simulink model "BackStepping"  (R2018b)
settings: Solver=VariableStepAuto  StartTime=0.0  StopTime=1  FixedStep=1  RelTol=0.1
values from neighbouring files (symbols this model uses):
  jointAngle = inverseKinematic.ComputeInverseKinematic(jointAngle, endPose)    [CartesianTrajectoryGeneration.m]
  jointAngleStart = [175.0; 145.0; 178.0; 90.0; 180.0; 215.0; 260.0]    [CartesianTrajectoryGeneration.m]
  K = [[100 0 0 0 0 0 0] ... (first row only)    [BackSteppingParam.m]
  Lamda = [[1 0 0 0 0 0 0] ... (first row only)    [BackSteppingParam.m]
settings Model: Creator=olavoie  LastModifiedBy=olavoie

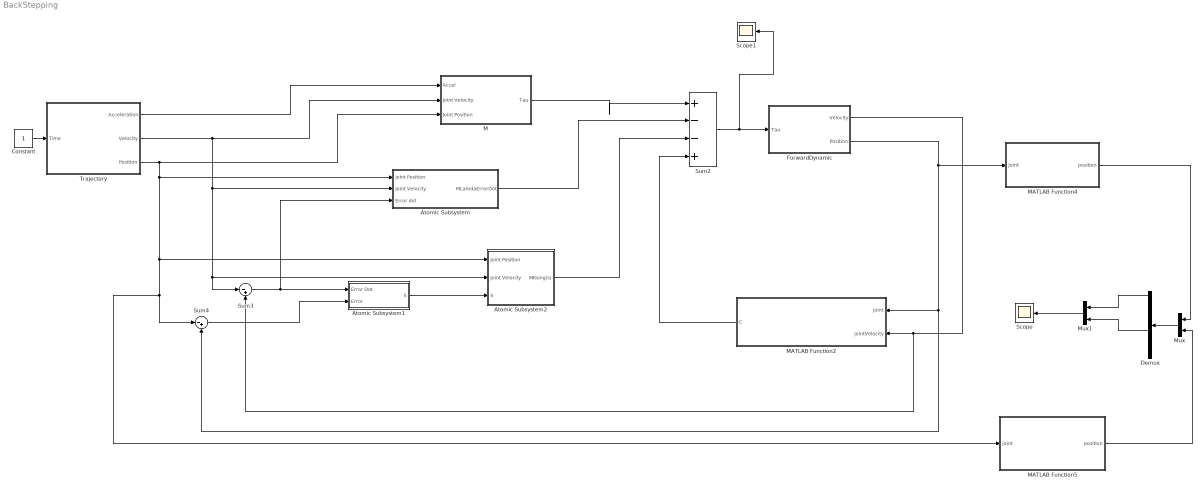
== system BackStepping ==
  Atomic Subsystem : Subsystem  TreatAsAtomicUnit=on
  Atomic Subsystem1 : Subsystem  TreatAsAtomicUnit=on
  Atomic Subsystem2 : Subsystem  TreatAsAtomicUnit=on
  Constant : Constant
  Demux : Demux  Outputs=6
  ForwardDynamic : Subsystem  TreatAsAtomicUnit=on
  M : Subsystem  TreatAsAtomicUnit=on
  MATLAB Function2 : MATLAB Function  TreatAsAtomicUnit=on
  MATLAB Function4 : MATLAB Function  TreatAsAtomicUnit=on
  MATLAB Function5 : MATLAB Function  TreatAsAtomicUnit=on
  Mux : Mux  Inputs=2
  Mux1 : Mux  Inputs=2
  Scope : Scope
  Scope1 : Scope
  Sum2 : Sum  Inputs=|+--+
  Sum3 : Sum  Inputs=|-+
  Sum4 : Sum  Inputs=|-+
  Trajectory : Subsystem  TreatAsAtomicUnit=on
  wires:
  Constant/1 -> Trajectory/1(Time)
  ForwardDynamic/1(Velocity) -> Sum3/2, MATLAB Function2/2(jointVelocity)
  Trajectory/1(Acceleration) -> M/1("Accel ")
  Trajectory/2(Velocity) -> Sum3/1, Atomic Subsystem2/2(Joint Velocity), Atomic Subsystem/2(Joint Velocity), M/2(Joint Velocity)
  Sum3/1 -> Atomic Subsystem/3(Error dot), Atomic Subsystem1/1(Error Dot)
  Sum4/1 -> Atomic Subsystem1/2(Error)
  Atomic Subsystem1/1(S) -> Atomic Subsystem2/3(S)
  Sum2/1 -> Scope1/1, ForwardDynamic/1(Tau)
  MATLAB Function2/1(C) -> Sum2/4
  M/1(Tau) -> Sum2/1
  MATLAB Function5/1(position) -> Mux/2
  MATLAB Function4/1(position) -> Mux/1
  ForwardDynamic/2(Position) -> Sum4/2, MATLAB Function2/1(joint), MATLAB Function4/1(joint)
  Trajectory/3(Position) -> Sum4/1, MATLAB Function5/1(joint), Atomic Subsystem2/1(Joint Position), Atomic Subsystem/1(Joint Position), M/3(Joint Position)
  Atomic Subsystem/1(MLamdaErrorDot) -> Sum2/2
  Atomic Subsystem2/1(MKsing(s)) -> Sum2/3
  Mux/1 -> Demux/1
  Demux/1 -> Mux1/1
  Demux/4 -> Mux1/2
  Mux1/1 -> Scope/1

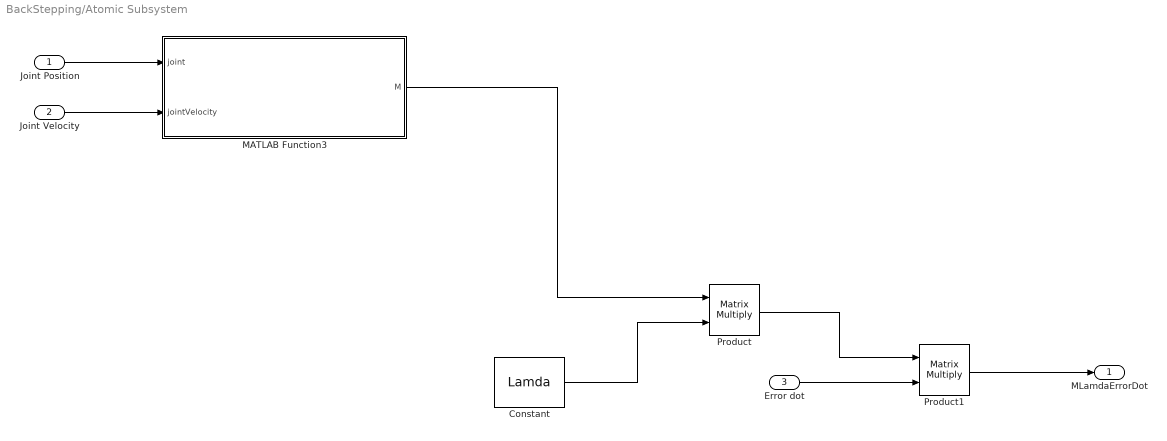
== system BackStepping/Atomic Subsystem ==
  Joint Position : Inport
  Joint Velocity : Inport  Port=2
  Error dot : Inport  Port=3
  Constant : Constant  Value=Lamda
  MATLAB Function3 : MATLAB Function  TreatAsAtomicUnit=on
  Product : Product  Multiplication=Matrix(*)
  Product1 : Product  Multiplication=Matrix(*)
  MLamdaErrorDot : Outport
  wires:
  Joint Position/1 -> MATLAB Function3/1(joint)
  Joint Velocity/1 -> MATLAB Function3/2(jointVelocity)
  Product1/1 -> MLamdaErrorDot/1
  Error dot/1 -> Product1/2
  Product/1 -> Product1/1
  Constant/1 -> Product/2
  MATLAB Function3/1(M) -> Product/1

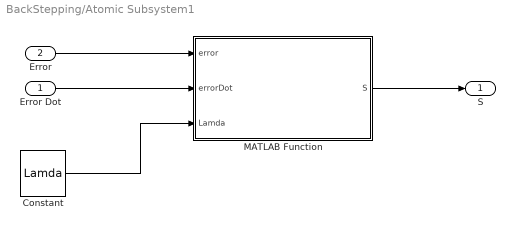
== system BackStepping/Atomic Subsystem1 ==
  Error Dot : Inport
  Error : Inport  Port=2
  Constant : Constant  Value=Lamda
  MATLAB Function : MATLAB Function  TreatAsAtomicUnit=on
  S : Outport
  wires:
  Error/1 -> MATLAB Function/1(error)
  Error Dot/1 -> MATLAB Function/2(errorDot)
  Constant/1 -> MATLAB Function/3(Lamda)
  MATLAB Function/1(S) -> S/1

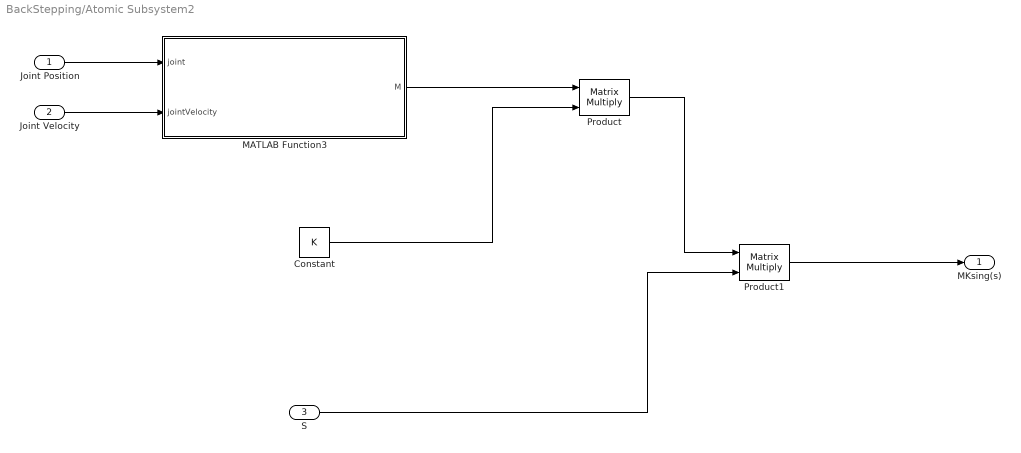
== system BackStepping/Atomic Subsystem2 ==
  Joint Position : Inport
  Joint Velocity : Inport  Port=2
  S : Inport  Port=3
  Constant : Constant  Value=K
  MATLAB Function3 : MATLAB Function  TreatAsAtomicUnit=on
  Product : Product  Multiplication=Matrix(*)
  Product1 : Product  Multiplication=Matrix(*)
  MKsing(s) : Outport
  wires:
  Joint Velocity/1 -> MATLAB Function3/2(jointVelocity)
  Joint Position/1 -> MATLAB Function3/1(joint)
  MATLAB Function3/1(M) -> Product/1
  Constant/1 -> Product/2
  Product/1 -> Product1/1
  Product1/1 -> MKsing(s)/1
  S/1 -> Product1/2

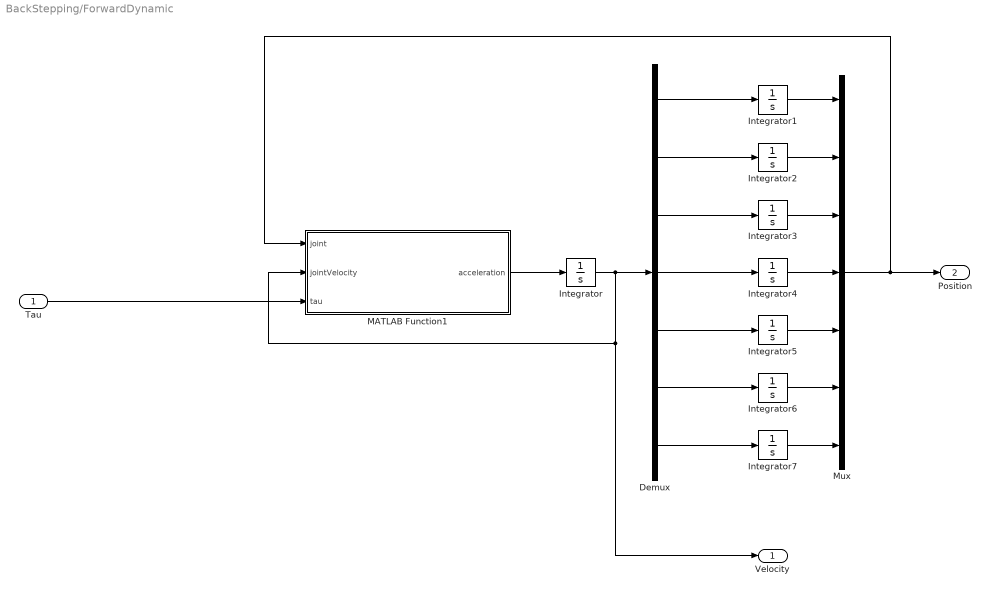
== system BackStepping/ForwardDynamic ==
  Tau : Inport
  Demux : Demux  Outputs=7
  Integrator : Integrator
  Integrator1 : Integrator  InitialCondition=jointAngleStart(1)
  Integrator2 : Integrator  InitialCondition=jointAngleStart(2)
  Integrator3 : Integrator  InitialCondition=jointAngleStart(3)
  Integrator4 : Integrator  InitialCondition=jointAngleStart(4)
  Integrator5 : Integrator  InitialCondition=jointAngleStart(5)
  Integrator6 : Integrator  InitialCondition=jointAngleStart(6)
  Integrator7 : Integrator  InitialCondition=jointAngleStart(7)
  MATLAB Function1 : MATLAB Function  TreatAsAtomicUnit=on
  Mux : Mux  Inputs=7
  Velocity : Outport
  Position : Outport  Port=2
  wires:
  Tau/1 -> MATLAB Function1/3(tau)
  MATLAB Function1/1(acceleration) -> Integrator/1
  Integrator/1 -> Velocity/1, MATLAB Function1/2(jointVelocity), Demux/1
  Demux/7 -> Integrator7/1
  Demux/6 -> Integrator6/1
  Demux/5 -> Integrator5/1
  Demux/4 -> Integrator4/1
  Demux/3 -> Integrator3/1
  Demux/1 -> Integrator1/1
  Demux/2 -> Integrator2/1
  Integrator1/1 -> Mux/1
  Integrator2/1 -> Mux/2
  Integrator3/1 -> Mux/3
  Integrator4/1 -> Mux/4
  Integrator5/1 -> Mux/5
  Integrator6/1 -> Mux/6
  Integrator7/1 -> Mux/7
  Mux/1 -> MATLAB Function1/1(joint), Position/1

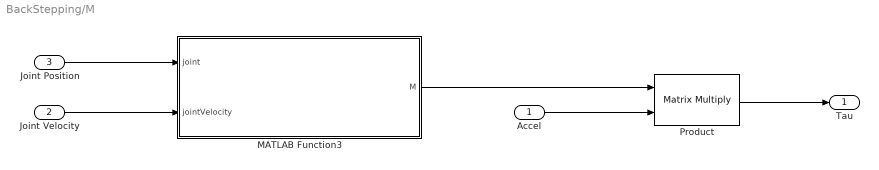
== system BackStepping/M ==
  "Accel " : Inport
  Joint Velocity : Inport  Port=2
  Joint Position : Inport  Port=3
  MATLAB Function3 : MATLAB Function  TreatAsAtomicUnit=on
  Product : Product  Multiplication=Matrix(*)
  Tau : Outport
  wires:
  MATLAB Function3/1(M) -> Product/1
  Product/1 -> Tau/1
  Joint Position/1 -> MATLAB Function3/1(joint)
  Joint Velocity/1 -> MATLAB Function3/2(jointVelocity)
  "Accel "/1 -> Product/2

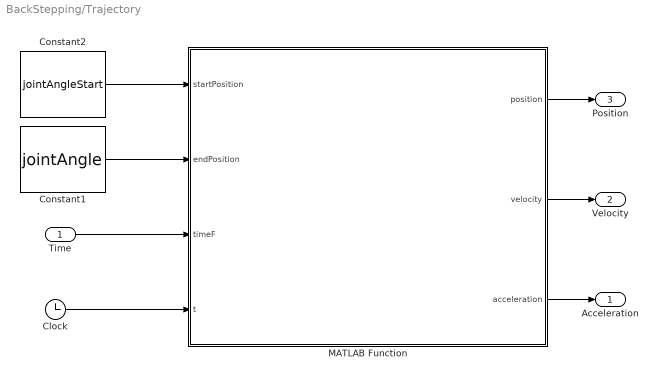
== system BackStepping/Trajectory ==
  Time : Inport
  Clock : Clock
  Constant1 : Constant  Value=jointAngle
  Constant2 : Constant  Value=jointAngleStart
  MATLAB Function : MATLAB Function  TreatAsAtomicUnit=on
  Acceleration : Outport
  Velocity : Outport  Port=2
  Position : Outport  Port=3
  wires:
  Constant1/1 -> MATLAB Function/2(endPosition)
  Time/1 -> MATLAB Function/3(timeF)
  Clock/1 -> MATLAB Function/4(t)
  Constant2/1 -> MATLAB Function/1(startPosition)
  MATLAB Function/1(position) -> Position/1
  MATLAB Function/2(velocity) -> Velocity/1
  MATLAB Function/3(acceleration) -> Acceleration/1

== matlab function BackStepping/M/MATLAB Function3 ==
  data: joint input; M output; jointVelocity input
function M = MassMatrix(joint, jointVelocity)
    % Robot Frame    
    robotData = RobotParam;
    
    % Mass Center
    Pc = zeros(3,7);
    Pc(:, 1) = [ -3.94e-06;  0.001804699;  -0.0748562];
    Pc(:, 2) = [2.2339e-05;   0.07515658;  -0.0301928];
    Pc(:, 3) = [-2.234e-05;  0.009582299;  -0.0966774];
    Pc(:, 4) = [-3.269e-05;   0.09546485;  -0.0287837];
    Pc(:, 5) = [6.4423e-05;  -0.00987523;  -0.0607337];
    Pc(:, 6) = [5.6819e-05;   0.04279498; -0.00982194];
    Pc(:, 7) = [         0;       -2e-05;    -0.01702];

    % Mass
    m = [1.290800 1.344200 1.344200 1.094520 0.590200 0.590200 0.239480];

    % Inertia
    I = zeros(3, 3,7);
    I(:, :, 1) = [101, 0, 0; 0, 101, 0; 0, 0, 101];
    I(:, :, 2) = [102, 0, 0; 0, 102, 0; 0, 0, 102];
    I(:, :, 3) = [103, 0, 0; 0, 103, 0; 0, 0, 103];
    I(:, :, 4) = [104, 0, 0; 0, 104, 0; 0, 0, 104];
    I(:, :, 5) = [105, 0, 0; 0, 105, 0; 0, 0, 105];
    I(:, :, 6) = [106, 0, 0; 0, 106, 0; 0, 0, 106];
    I(:, :, 7) = [107, 0, 0; 0, 107, 0; 0, 0, 107];

    R = zeros(3, 3, robotData.mActuatorCount + 1);
    P = zeros(3, robotData.mActuatorCount + 1);

    % Robot referential
    for n = 1:robotData.mActuatorCount
        T = robotData.mJointReferentiel(:, :, n) * rotm2tform(rotz(joint(n) + robotData.mJointOffset(n)));
        R(:, :, n) = tform2rotm(T);
        P(:, n)    = tform2trvec(T);
    end
    
    R(:, :, robotData.mActuatorCount + 1) = [1, 0, 0; 0, 1, 0; 0, 1, 0];
    P(:, robotData.mActuatorCount + 1)    = [0; 0; 0];

    C = InverseDynamicSolver(R, P, Pc, I, m, jointVelocity, [0; 0; 0; 0; 0; 0; 0; 0], robotData.mActuatorCount)';

    M = zeros(7,7);
    for n = 1:robotData.mActuatorCount
        a = [0; 0; 0; 0; 0; 0; 0];
        a(n) = 1;
        M(:, n) = InverseDynamicSolver(R, P, Pc, I, m, jointVelocity, a, robotData.mActuatorCount)' - C;
    end 
end

== matlab function BackStepping/Atomic Subsystem/MATLAB Function3 ==
  data: joint input; M output; jointVelocity input
function M = MassMatrix(joint, jointVelocity)
    % Robot Frame    
    robotData = RobotParam;
    
    % Mass Center
    Pc = zeros(3,7);
    Pc(:, 1) = [ -3.94e-06;  0.001804699;  -0.0748562];
    Pc(:, 2) = [2.2339e-05;   0.07515658;  -0.0301928];
    Pc(:, 3) = [-2.234e-05;  0.009582299;  -0.0966774];
    Pc(:, 4) = [-3.269e-05;   0.09546485;  -0.0287837];
    Pc(:, 5) = [6.4423e-05;  -0.00987523;  -0.0607337];
    Pc(:, 6) = [5.6819e-05;   0.04279498; -0.00982194];
    Pc(:, 7) = [         0;       -2e-05;    -0.01702];

    % Mass
    m = [1.290800 1.344200 1.344200 1.094520 0.590200 0.590200 0.239480];

    % Inertia
    I = zeros(3, 3,7);
    I(:, :, 1) = [101, 0, 0; 0, 101, 0; 0, 0, 101];
    I(:, :, 2) = [102, 0, 0; 0, 102, 0; 0, 0, 102];
    I(:, :, 3) = [103, 0, 0; 0, 103, 0; 0, 0, 103];
    I(:, :, 4) = [104, 0, 0; 0, 104, 0; 0, 0, 104];
    I(:, :, 5) = [105, 0, 0; 0, 105, 0; 0, 0, 105];
    I(:, :, 6) = [106, 0, 0; 0, 106, 0; 0, 0, 106];
    I(:, :, 7) = [107, 0, 0; 0, 107, 0; 0, 0, 107];

    R = zeros(3, 3, robotData.mActuatorCount + 1);
    P = zeros(3, robotData.mActuatorCount + 1);

    % Robot referential
    for n = 1:robotData.mActuatorCount
        T = robotData.mJointReferentiel(:, :, n) * rotm2tform(rotz(joint(n) + robotData.mJointOffset(n)));
        R(:, :, n) = tform2rotm(T);
        P(:, n)    = tform2trvec(T);
    end
    
    R(:, :, robotData.mActuatorCount + 1) = [1, 0, 0; 0, 1, 0; 0, 1, 0];
    P(:, robotData.mActuatorCount + 1)    = [0; 0; 0];

    C = InverseDynamicSolver(R, P, Pc, I, m, jointVelocity, [0; 0; 0; 0; 0; 0; 0; 0], robotData.mActuatorCount)';

    M = zeros(7,7);
    for n = 1:robotData.mActuatorCount
        a = [0; 0; 0; 0; 0; 0; 0];
        a(n) = 1;
        M(:, n) = InverseDynamicSolver(R, P, Pc, I, m, jointVelocity, a, robotData.mActuatorCount)' - C;
    end 
end

== matlab function BackStepping/MATLAB Function2 ==
  data: joint input; C output; jointVelocity input
function C = SystemCompensation(joint, jointVelocity)
    % Robot Frame
    acceleration = zeros(size(jointVelocity));
    
    robotData = RobotParam;
    
    % Mass Center
    Pc = zeros(3,7);
    Pc(:, 1) = [ -3.94e-06;  0.001804699;  -0.0748562];
    Pc(:, 2) = [2.2339e-05;   0.07515658;  -0.0301928];
    Pc(:, 3) = [-2.234e-05;  0.009582299;  -0.0966774];
    Pc(:, 4) = [-3.269e-05;   0.09546485;  -0.0287837];
    Pc(:, 5) = [6.4423e-05;  -0.00987523;  -0.0607337];
    Pc(:, 6) = [5.6819e-05;   0.04279498; -0.00982194];
    Pc(:, 7) = [         0;       -2e-05;    -0.01702];

    % Mass
    m = [1.290800 1.344200 1.344200 1.094520 0.590200 0.590200 0.239480];

    % Inertia
    I = zeros(3, 3,7);
    I(:, :, 1) = [101, 0, 0; 0, 101, 0; 0, 0, 101];
    I(:, :, 2) = [102, 0, 0; 0, 102, 0; 0, 0, 102];
    I(:, :, 3) = [103, 0, 0; 0, 103, 0; 0, 0, 103];
    I(:, :, 4) = [104, 0, 0; 0, 104, 0; 0, 0, 104];
    I(:, :, 5) = [105, 0, 0; 0, 105, 0; 0, 0, 105];
    I(:, :, 6) = [106, 0, 0; 0, 106, 0; 0, 0, 106];
    I(:, :, 7) = [107, 0, 0; 0, 107, 0; 0, 0, 107];

    R = zeros(3, 3, robotData.mActuatorCount + 1);
    P = zeros(3, robotData.mActuatorCount + 1);

    % Robot referential
    for n = 1:robotData.mActuatorCount
        T = robotData.mJointReferentiel(:, :, n) * rotm2tform(rotz(joint(n) + robotData.mJointOffset(n)));
        R(:, :, n) = tform2rotm(T);
        P(:, n)    = tform2trvec(T);
    end
    
    R(:, :, robotData.mActuatorCount + 1) = [1, 0, 0; 0, 1, 0; 0, 1, 0];
    P(:, robotData.mActuatorCount + 1)    = [0; 0; 0];

    C = InverseDynamicSolver(R, P, Pc, I, m, jointVelocity, [0; 0; 0; 0; 0; 0; 0; 0], robotData.mActuatorCount)';
end

== matlab function BackStepping/ForwardDynamic/MATLAB Function1 ==
  data: joint input; acceleration output; jointVelocity input; tau input
function acceleration = ForwardDynamicSolver(joint, jointVelocity, tau)
    % Robot Frame
    acceleration = zeros(7, 1);
    
    robotData = RobotParam;
    
    % Mass Center
    Pc = zeros(3,7);
    Pc(:, 1) = [ -3.94e-06;  0.001804699;  -0.0748562];
    Pc(:, 2) = [2.2339e-05;   0.07515658;  -0.0301928];
    Pc(:, 3) = [-2.234e-05;  0.009582299;  -0.0966774];
    Pc(:, 4) = [-3.269e-05;   0.09546485;  -0.0287837];
    Pc(:, 5) = [6.4423e-05;  -0.00987523;  -0.0607337];
    Pc(:, 6) = [5.6819e-05;   0.04279498; -0.00982194];
    Pc(:, 7) = [         0;       -2e-05;    -0.01702];

    % Mass
    m = [3.290800 3.344200 3.344200 3.094520 3.590200 3.590200 3.239480];

    % Inertia
    I = zeros(3, 3, 7);
    I(:, :, 1) = [101, 0, 0; 0, 101, 0; 0, 0, 101];
    I(:, :, 2) = [102, 0, 0; 0, 102, 0; 0, 0, 102];
    I(:, :, 3) = [103, 0, 0; 0, 103, 0; 0, 0, 103];
    I(:, :, 4) = [104, 0, 0; 0, 104, 0; 0, 0, 104];
    I(:, :, 5) = [105, 0, 0; 0, 105, 0; 0, 0, 105];
    I(:, :, 6) = [106, 0, 0; 0, 106, 0; 0, 0, 106];
    I(:, :, 7) = [107, 0, 0; 0, 107, 0; 0, 0, 107];

    R = zeros(3, 3, robotData.mActuatorCount + 1);
    P = zeros(3, robotData.mActuatorCount + 1);

    % Robot referential
    for n = 1:robotData.mActuatorCount
        T = robotData.mJointReferentiel(:, :, n) * rotm2tform(rotz(joint(n) + robotData.mJointOffset(n)));
        R(:, :, n) = tform2rotm(T);
        P(:, n)    = tform2trvec(T);
    end
    
    R(:, :, robotData.mActuatorCount + 1) = [1, 0, 0; 0, 1, 0; 0, 1, 0];
    P(:, robotData.mActuatorCount + 1)    = [0; 0; 0];

    C = InverseDynamicSolver(R, P, Pc, I, m, jointVelocity, [0; 0; 0; 0; 0; 0; 0; 0], robotData.mActuatorCount)';

    M = zeros(7,7);
    for n = 1:robotData.mActuatorCount
        a = [0; 0; 0; 0; 0; 0; 0];
        a(n) = 1;
        M(:, n) = InverseDynamicSolver(R, P, Pc, I, m, jointVelocity, a, robotData.mActuatorCount)' - C;
    end 
    acceleration(:, 1) = inv(M) * (tau - C);
end

== matlab function BackStepping/Atomic Subsystem2/MATLAB Function3 ==
  data: joint input; M output; jointVelocity input
function M = MassMatrix(joint, jointVelocity)
    % Robot Frame    
    robotData = RobotParam;
    
    % Mass Center
    Pc = zeros(3,7);
    Pc(:, 1) = [ -3.94e-06;  0.001804699;  -0.0748562];
    Pc(:, 2) = [2.2339e-05;   0.07515658;  -0.0301928];
    Pc(:, 3) = [-2.234e-05;  0.009582299;  -0.0966774];
    Pc(:, 4) = [-3.269e-05;   0.09546485;  -0.0287837];
    Pc(:, 5) = [6.4423e-05;  -0.00987523;  -0.0607337];
    Pc(:, 6) = [5.6819e-05;   0.04279498; -0.00982194];
    Pc(:, 7) = [         0;       -2e-05;    -0.01702];

    % Mass
    m = [1.290800 1.344200 1.344200 1.094520 0.590200 0.590200 0.239480];

    % Inertia
    I = zeros(3, 3,7);
    I(:, :, 1) = [101, 0, 0; 0, 101, 0; 0, 0, 101];
    I(:, :, 2) = [102, 0, 0; 0, 102, 0; 0, 0, 102];
    I(:, :, 3) = [103, 0, 0; 0, 103, 0; 0, 0, 103];
    I(:, :, 4) = [104, 0, 0; 0, 104, 0; 0, 0, 104];
    I(:, :, 5) = [105, 0, 0; 0, 105, 0; 0, 0, 105];
    I(:, :, 6) = [106, 0, 0; 0, 106, 0; 0, 0, 106];
    I(:, :, 7) = [107, 0, 0; 0, 107, 0; 0, 0, 107];

    R = zeros(3, 3, robotData.mActuatorCount + 1);
    P = zeros(3, robotData.mActuatorCount + 1);

    % Robot referential
    for n = 1:robotData.mActuatorCount
        T = robotData.mJointReferentiel(:, :, n) * rotm2tform(rotz(joint(n) + robotData.mJointOffset(n)));
        R(:, :, n) = tform2rotm(T);
        P(:, n)    = tform2trvec(T);
    end
    
    R(:, :, robotData.mActuatorCount + 1) = [1, 0, 0; 0, 1, 0; 0, 1, 0];
    P(:, robotData.mActuatorCount + 1)    = [0; 0; 0];

    C = InverseDynamicSolver(R, P, Pc, I, m, jointVelocity, [0; 0; 0; 0; 0; 0; 0; 0], robotData.mActuatorCount)';

    M = zeros(7,7);
    for n = 1:robotData.mActuatorCount
        a = [0; 0; 0; 0; 0; 0; 0];
        a(n) = 1;
        M(:, n) = InverseDynamicSolver(R, P, Pc, I, m, jointVelocity, a, robotData.mActuatorCount)' - C;
    end 
end

== matlab function BackStepping/MATLAB Function4 ==
  data: joint input; position output
function position = ForwardKinematic(joint)
    position = [0,0,0];
    frame = zeros(4,4,7);
    mRobotParam = RobotParam;
            
    frame(:, :, 1) = mRobotParam.mJointReferentiel(:, :, 1) * rotm2tform(rotz(joint(1) + mRobotParam.mJointOffset(1)));
    
    for n = 2:mRobotParam.mActuatorCount
        frame(:, :, n) = frame(:, :, n - 1) * mRobotParam.mJointReferentiel(:, :, n) * rotm2tform(rotz(joint(n) + mRobotParam.mJointOffset(n)));
    end
    
    position = tform2trvec(frame(:, :, mRobotParam.mActuatorCount));

== matlab function BackStepping/Trajectory/MATLAB Function ==
  data: startPosition input; position output; endPosition input; timeF input; t input; velocity output; acceleration output
function  [position, velocity, acceleration] = Trajectory(startPosition, endPosition, timeF, t)

    position = zeros(size(startPosition));
    velocity = zeros(size(startPosition));
    acceleration = zeros(size(startPosition));
    
    if t >= timeF
        t = timeF;
    end

    for i = 1:length(startPosition)    
        S      = [startPosition(i); 0; 0; endPosition(i); 0; 0];
        M      = [1 0 0 0 0 0; 0 1 0 0 0 0; 0 0 2 0 0 0; 1 timeF timeF^2 timeF^3 timeF^4 timeF^5; 0 1 2*timeF 3*timeF^2 4*timeF^3 5*timeF^4; 0 0 2 (3*2)*timeF 4*3*timeF^2 5*4*timeF^3];

        a = M^-1 * S;
        
        position(i)     = a(1) + a(2) * t + a(3) * t^2 + a(4) * t^3 + a(5) * t^4 + a(6) * t^5;
        velocity(i)     = a(2) + 2 * a(3) * t + 3 * a(4) * t^2 + 4 * a(5) * t^3 + 5 * a(6) * t^4;
        acceleration(i) = 2 * a(3) + (3 * 2) * a(4) * t + (4 * 3) * a(5) * t^2 + (4 * 5) * a(6) * t^3;
    end

== matlab function BackStepping/MATLAB Function5 ==
  data: joint input; position output
function position = ForwardKinematic(joint)
    position = [0,0,0];
    frame = zeros(4,4,7);
    mRobotParam = RobotParam;
            
    frame(:, :, 1) = mRobotParam.mJointReferentiel(:, :, 1) * rotm2tform(rotz(joint(1) + mRobotParam.mJointOffset(1)));
    
    for n = 2:mRobotParam.mActuatorCount
        frame(:, :, n) = frame(:, :, n - 1) * mRobotParam.mJointReferentiel(:, :, n) * rotm2tform(rotz(joint(n) + mRobotParam.mJointOffset(n)));
    end
    
    position = tform2trvec(frame(:, :, mRobotParam.mActuatorCount));

== matlab function BackStepping/Atomic Subsystem1/MATLAB Function ==
  data: error input; S output; errorDot input; Lamda input
function S = ComputeS(error, errorDot, Lamda)
    S = Lamda*error + errorDot;
